simulink model "kinematicModel"  (R2022a)
settings: Solver=ode4  StartTime=0.0  StopTime=10  FixedStep=0.01  RelTol=1e-3  EnableMultiTasking=on
values from neighbouring files (symbols this model uses):
  x0 = op.States.x    [cal_trim_durumi2.m]
undefined symbols (not defined in the file or in its folder): e0_0, e1_0, e2_0, e3_0
libraries: simulink_extras x3, sharedtransform x3
settings Model: Creator=김응태  LastModifiedBy=USer
settings DataIOCC: ExternalInput=[0 -0.0167603073066386 -9.24526122738572e-06 0.000171264505376752 0.751623301103014]  InitialState=[]  LimitDataPoints=on  SaveFormat=Array  SignalLoggingSaveFormat=ModelDataLogs  ReturnWorkspaceOutputs=off  SignalLoggingName=sigsOut
settings OptimizationCC: DefaultParameterBehavior=Inlined  BufferReuse=off
settings DebuggingCC: SaveWithParameterizedLinksMsg=none  MergeDetectMultiDrivingBlocksExec=none  SignalResolutionControl=TryResolveAllWithWarning  MultiTaskDSMMsg=warning  MultiTaskCondExecSysMsg=none  UnconnectedInputMsg=warning  UnconnectedOutputMsg=warning  UnconnectedLineMsg=warning  InitInArrayFormatMsg=none
settings HardwareCC: ProdBitPerPointer=32  ProdBitPerSizeT=32  ProdBitPerPtrDiffT=32  ProdLargestAtomicFloat=None  ProdIntDivRoundTo=Undefined  ProdEndianess=Unspecified  ProdWordSize=32  ProdHWDeviceType=32-bit Generic  TargetUnknown=on
settings ModelReferenceCC: PropagateSignalLabelsOutOfModel=off
settings GRTTargetCC: CombineOutputUpdateFcns=off  GRTInterface=on
settings ConfigComp: CovMetricSettings=dw  CovSaveCumulativeToWorkspaceVar=on  CovSaveSingleToWorkspaceVar=on

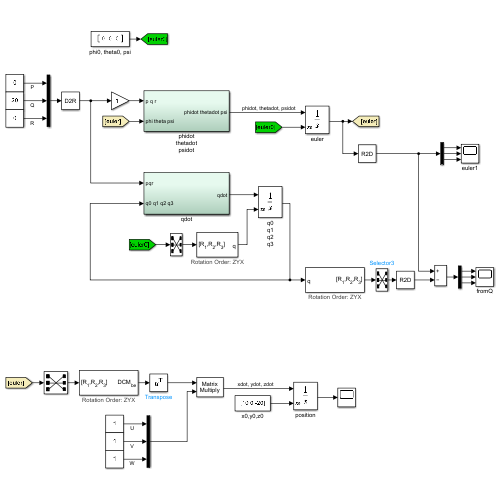
[thumbnail: Simulink's stored preview of the top-level diagram]
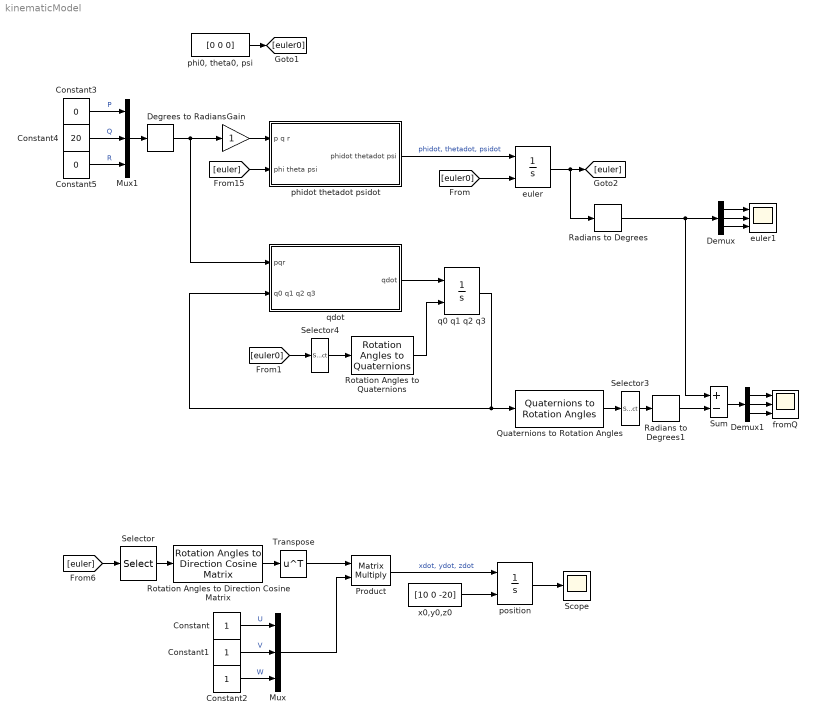
== system kinematicModel ==
  Constant : Constant
  Constant1 : Constant
  Constant2 : Constant
  Constant3 : Constant  Value=0
  Constant4 : Constant  Value=20
  Constant5 : Constant  Value=0
  Degrees to Radians : simulink_extras/Transformations/Degrees to Radians
  Demux : Demux  Outputs=3
  Demux1 : Demux  Outputs=3
  Gain : Gain
  Mux : Mux  Inputs=3
  Mux1 : Mux  Inputs=3
  Product : Product  Multiplication=Matrix(*)  InputSameDT=on  RndMeth=Zero  SaturateOnIntegerOverflow=on  OutDataTypeStr=Inherit: Same as first input
  Quaternions to Rotation Angles : sharedtransform/Quaternions to Rotation Angles  rotationOrder=ZYX  aMode=aMode
      settings: SourceProductBaseCode=AE,PW,DR,MT,VE
  Radians to Degrees : simulink_extras/Transformations/Radians to Degrees
  Radians to Degrees1 : simulink_extras/Transformations/Radians to Degrees
  Rotation Angles to Direction Cosine Matrix : sharedtransform/Rotation Angles to Direction Cosine Matrix  rotationOrder=ZYX  aMode=aMode
      settings: SourceProductBaseCode=AE,PW,DR,MT,VE
  Rotation Angles to Quaternions : sharedtransform/Rotation Angles to Quaternions  rotationOrder=ZYX  aMode=aMode
      settings: SourceProductBaseCode=AE,PW,DR,MT,VE
  Scope : Scope
  Selector : Selector  InputPortWidth=3  IndexOptions=Index vector (dialog)  Indices=[3 2 1]  OutputSizes=1
  Selector3 : Selector  InputPortWidth=3  IndexOptions=Index vector (dialog)  Indices=[3 2 1]  OutputSizes=1
  Selector4 : Selector  InputPortWidth=3  IndexOptions=Index vector (dialog)  Indices=[3 2 1]  OutputSizes=1
  Sum : Sum  Inputs=+-
  Transpose : Math  Operator=transpose  SignedPower=on
  euler : Integrator  InitialConditionSource=external  InitialCondition=x0
  euler1 : Scope  NumInputPorts=3
  fromQ : Scope  NumInputPorts=3
  "phi0, theta0, psi" : Constant  Value=[0 0 0]
  phidot thetadot psidot : Subsystem  AncestorBlock=|
      | aerolib6dofsys/DCM & Euler Angles (Euler)/phidot
      | thetadot
      | psidot
  position : Integrator  InitialConditionSource=external  InitialCondition=x0
  q0 q1 q2 q3 : Integrator  InitialConditionSource=external  InitialCondition=[e0_0 e1_0 e2_0 e3_0]  ContinuousStateAttributes="\"\""
  qdot : Subsystem  AncestorBlock=|
      | aerolib6dofsys/DCM & Euler Angles (Euler)/phidot
      | thetadot
      | psidot
  x0,y0,z0 : Constant  Value=[10 0 -20]
  wires:
  phidot thetadot psidot/1(phidot thetadot psi) -> euler/1  "phidot, thetadot, psidot"
  [euler] -> phidot thetadot psidot/2(phi theta psi)
  Product/1 -> position/1  "xdot, ydot, zdot"
  [euler0] -> euler/2
  Mux/1 -> Product/2
  x0,y0,z0/1 -> position/2
  euler/1 -> Radians to Degrees/1, [euler]
  position/1 -> Scope/1
  Radians to Degrees/1 -> Sum/1, Demux/1
  Degrees to Radians/1 -> qdot/1(pqr), Gain/1
  Constant/1 -> Mux/1  "U"
  Constant1/1 -> Mux/2  "V"
  Constant2/1 -> Mux/3  "W"
  Constant5/1 -> Mux1/3  "R"
  Constant4/1 -> Mux1/2  "Q"
  Constant3/1 -> Mux1/1  "P"
  Gain/1 -> phidot thetadot psidot/1(p q r)
  Selector/1 -> Rotation Angles to Direction Cosine Matrix/1
  Rotation Angles to Direction Cosine Matrix/1 -> Transpose/1
  Transpose/1 -> Product/1
  [euler] -> Selector/1
  [euler0] -> Selector4/1
  qdot/1(qdot) -> q0 q1 q2 q3/1
  q0 q1 q2 q3/1 -> qdot/2(q0 q1 q2 q3), Quaternions to Rotation Angles/1
  Mux1/1 -> Degrees to Radians/1
  Selector4/1 -> Rotation Angles to Quaternions/1
  Rotation Angles to Quaternions/1 -> q0 q1 q2 q3/2
  Quaternions to Rotation Angles/1 -> Selector3/1
  Selector3/1 -> Radians to Degrees1/1
  "phi0, theta0, psi"/1 -> [euler0]
  Demux1/1 -> fromQ/1
  Demux1/2 -> fromQ/2
  Demux1/3 -> fromQ/3
  Demux/1 -> euler1/1
  Demux/2 -> euler1/2
  Demux/3 -> euler1/3
  Radians to Degrees1/1 -> Sum/2
  Sum/1 -> Demux1/1

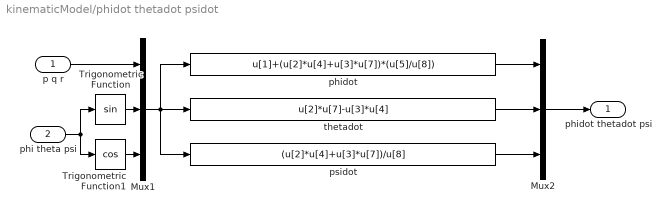
== system kinematicModel/phidot thetadot psidot ==
  p q r : Inport
  phi theta psi : Inport  Port=2
  Mux1 : Mux  Inputs=[3 3 3]
  Mux2 : Mux  Inputs=3
  Trigonometric Function : Trigonometry
  Trigonometric Function1 : Trigonometry  Operator=cos
  phidot : Fcn  Expr=u[1]+(u[2]*u[4]+u[3]*u[7])*(u[5]/u[8])
  psidot : Fcn  Expr=(u[2]*u[4]+u[3]*u[7])/u[8]
  thetadot : Fcn  Expr=u[2]*u[7]-u[3]*u[4]
  phidot thetadot psi : Outport  InitialOutput=0  VectorParamsAs1DForOutWhenUnconnected=off
  wires:
  Trigonometric Function1/1 -> Mux1/3
  Trigonometric Function/1 -> Mux1/2
  Mux2/1 -> phidot thetadot psi/1
  phidot/1 -> Mux2/1
  thetadot/1 -> Mux2/2
  psidot/1 -> Mux2/3
  phi theta psi/1 -> Trigonometric Function1/1, Trigonometric Function/1
  p q r/1 -> Mux1/1
  Mux1/1 -> thetadot/1, phidot/1, psidot/1

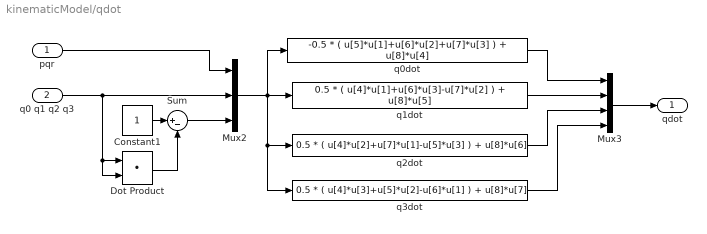
== system kinematicModel/qdot ==
  pqr : Inport
  q0 q1 q2 q3 : Inport  Port=2
  Constant1 : Constant
  Dot Product : DotProduct  InputSameDT=off  OutDataTypeStr=Inherit: Inherit via internal rule
  Mux2 : Mux  Inputs=[3 4 1]
  Mux3 : Mux
  Sum : Sum  Inputs=|+-  InputSameDT=on  SaturateOnIntegerOverflow=on  OutDataTypeStr=Inherit: Same as first input
  q0dot : Fcn  Expr=-0.5 * ( u[5]*u[1]+u[6]*u[2]+u[7]*u[3] ) + u[8]*u[4]
  q1dot : Fcn  Expr=0.5 * ( u[4]*u[1]+u[6]*u[3]-u[7]*u[2] ) + u[8]*u[5]
  q2dot : Fcn  Expr=0.5 * ( u[4]*u[2]+u[7]*u[1]-u[5]*u[3] ) + u[8]*u[6]
  q3dot : Fcn  Expr=0.5 * ( u[4]*u[3]+u[5]*u[2]-u[6]*u[1] ) + u[8]*u[7]
  qdot : Outport
  wires:
  q1dot/1 -> Mux3/2
  q0 q1 q2 q3/1 -> Mux2/2, Dot Product/2, Dot Product/1
  Sum/1 -> Mux2/3
  Dot Product/1 -> Sum/2
  q0dot/1 -> Mux3/1
  Mux3/1 -> qdot/1
  Mux2/1 -> q1dot/1, q0dot/1, q3dot/1, q2dot/1
  q2dot/1 -> Mux3/3
  q3dot/1 -> Mux3/4
  Constant1/1 -> Sum/1
  pqr/1 -> Mux2/1
